simulink model "attitude_controller"  (R2016a)
settings: Solver=VariableStepAuto  StartTime=0.0  StopTime=10.0  RelTol=1e-3
settings Model: Creator=anne  LastModifiedBy=anne
settings GRTTargetCC: GeneratePreprocessorConditionals=Use local settings

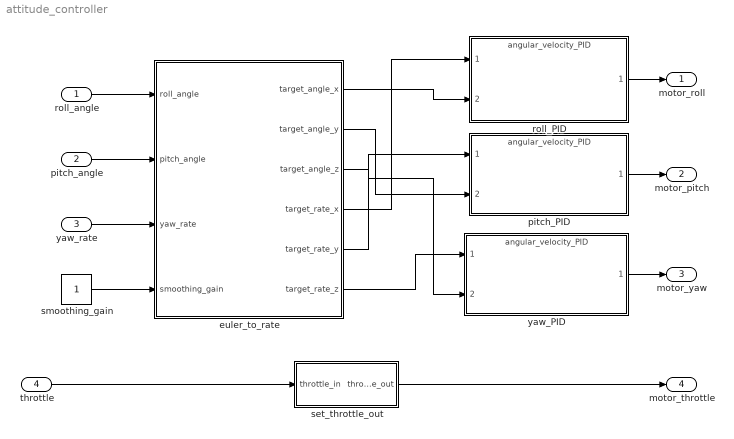
== system attitude_controller ==
  roll_angle : Inport
  pitch_angle : Inport  Port=2
  yaw_rate : Inport  Port=3
  throttle : Inport  Port=4
  euler_to_rate : Subsystem
  pitch_PID : ModelReference  ModelNameDialog=angular_velocity_PID.slx  SimulationMode=Normal  ModelReferenceVersion=1.2
  roll_PID : ModelReference  ModelNameDialog=angular_velocity_PID.slx  SimulationMode=Normal  ModelReferenceVersion=1.2
  set_throttle_out : Subsystem
  smoothing_gain : Constant
  yaw_PID : ModelReference  ModelNameDialog=angular_velocity_PID.slx  SimulationMode=Normal  ModelReferenceVersion=1.2
  motor_roll : Outport
  motor_pitch : Outport  Port=2
  motor_yaw : Outport  Port=3
  motor_throttle : Outport  Port=4
  wires:
  throttle/1 -> set_throttle_out/1(throttle_in)
  roll_angle/1 -> euler_to_rate/1(roll_angle)
  pitch_angle/1 -> euler_to_rate/2(pitch_angle)
  yaw_rate/1 -> euler_to_rate/3(yaw_rate)
  smoothing_gain/1 -> euler_to_rate/4(smoothing_gain)
  set_throttle_out/1(throttle_out) -> motor_throttle/1
  yaw_PID/1 -> motor_yaw/1
  pitch_PID/1 -> motor_pitch/1
  roll_PID/1 -> motor_roll/1
  euler_to_rate/1(target_angle_x) -> roll_PID/2
  euler_to_rate/4(target_rate_x) -> roll_PID/1
  euler_to_rate/2(target_angle_y) -> pitch_PID/2
  euler_to_rate/5(target_rate_y) -> pitch_PID/1
  euler_to_rate/6(target_rate_z) -> yaw_PID/1
  euler_to_rate/3(target_angle_z) -> yaw_PID/2

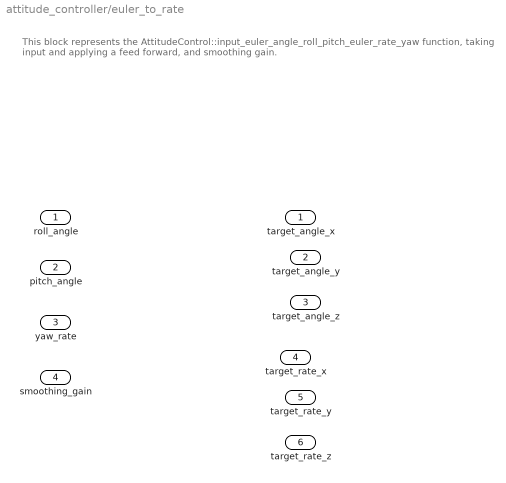
== system attitude_controller/euler_to_rate ==
  note: This block represents the AttitudeControl::input_euler_angle_roll_pitch_euler_rate_yaw function, taking input and applying a feed forward, and smoothing gain.
  roll_angle : Inport
  pitch_angle : Inport  Port=2
  yaw_rate : Inport  Port=3
  smoothing_gain : Inport  Port=4
  target_angle_x : Outport
  target_angle_y : Outport  Port=2
  target_angle_z : Outport  Port=3
  target_rate_x : Outport  Port=4
  target_rate_y : Outport  Port=5
  target_rate_z : Outport  Port=6

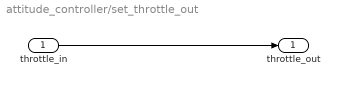
== system attitude_controller/set_throttle_out ==
  throttle_in : Inport
  throttle_out : Outport
  wires:
  throttle_in/1 -> throttle_out/1
